simulink model "Main_EntryPoint"  (R2024b)
settings: Solver=VariableStepAuto  StartTime=0.0  StopTime=10.0  RelTol=1e-3
(part 2 of 2)

== stateflow chart Main_EntryPoint/Chart ==
  state Main_EntryPoint1 [parallel]
    Main_EntryPoint()
    settings: executionOrder=1
  data: i_byBlockDirectionId function_input uint8; i_stBlockDirectionData function_input Bus: ST_BlockDirection; staBlockDirectionAy temporary Bus: ST_BlockDirection size=8; o_stRegionData function_output Bus: ST_ShuntingRegionTable; i_byRegionId function_input uint8; i_staShuntingRegionArray function_input Bus: ST_ShuntingRegion size=16; stShuntingRegionData temporary Bus: ST_ShuntingRegion; i_byRegionId function_input BYTE; o_stRegionData function_output Bus: ST_MaintenanceRegion size=1; i_byRegionId function_input uint8; o_bResult function_output boolean; stTableData temporary Bus: ST_ShuntingRegionTable; i_byRegionId function_input BYTE; i_staRegionDataArray function_input Bus: ST_MaintenanceRegion size=16; o_stRegionData function_output Bus: ST_MaintenanceRegion; i_byShuntingId function_input BYTE; i_stShuntingData function_input Bus: ST_ShuntingRegion; i_byBlockDirectionId function_input uint8; i_stBlockDirectionData function_input Bus: ST_BlockDirection; i_staBlockDirectionArray function_input Bus: ST_BlockDirection size=8; o_staBlockDirectionArray function_output Bus: ST_BlockDirection size=8; i_byRegionId function_input uint8; i_staRegionArray function_input Bus: ST_ShuntingRegionTable size=16; o_stRegionData function_output Bus: ST_ShuntingRegionTable; i_staTableDataArray function_input Bus: ST_InterlockingTrackLock size=8; o_bResult function_output BOOL; o_bResult function_output BOOL; i_byRegionId function_input BYTE; i_byRegionId function_input BYTE; i_stRegionData function_input Bus: ST_ShuntingRegion; i_staShuntingRegionArray function_input Bus: ST_ShuntingRegion size=16; o_staShuntingRegionArray function_output Bus: ST_ShuntingRegion size=16; i_staTableDataArray function_input Bus: ST_InterlockingRouteCheck size=24; o_bResult function_output BOOL; i_byBlockDirectionId function_input uint8; i_bStatus function_input boolean; stBlockDirectionData temporary Bus: ST_BlockDirection; i_staTableDataArray function_input Bus: ST_InterlockingPointMachineCheck size=12; o_bResult function_output BOOL; i_byRegionId function_input uint8; o_bResult function_output BOOL; stRegionData temporary Bus: ST_MaintenanceRegion; i_byRegionId function_input BYTE; o_stRegionData function_output Bus: ST_ShuntingRegion; i_staTableDataArray function_input Bus: ST_InterlockingPointMachineCheck size=12; o_bResult function_output BOOL; i_byBlockDirectionId function_input BYTE; o_bResult function_output BOOL; i_staTableDataArray function_input Bus: ST_InterlockingRouteCheck size=24; o_bResult function_output BOOL; i_byRegionId function_input BYTE; i_staShuntingRegionArray function_input Bus: ST_ShuntingRegion size=16; o_stRegionData function_output Bus: ST_ShuntingRegion; i_staTableDataArray function_input Bus: ST_InterlockingSignalCheck size=8; o_bResult function_output BOOL; i_byBlockDirectionId function_input uint8; o_stBlockDirectionData function_output Bus: ST_BlockDirection; i_iType function_input INT; i_ID function_input BYTE; o_bIsCheckID function_output boolean; i_byRegionId function_input uint8; o_bResult function_output boolean; o_aLevelCrossingSetPowerAy function_output BOOL size=8; i_stCmd function_input Bus: ST_IXLCommand; stShuntingRegionTableData temporary Bus: ST_ShuntingRegionTable; i_byRegionId function_input uint8; o_IsExist function_output boolean; i_byBlockDirectionId function_input uint8; i_staBlockDirectionArray function_input Bus: ST_BlockDirection size=8; o_stBlockDirectionData function_output Bus: ST_BlockDirection; o_aPMSetNormalAy function_output BOOL size=36; o_aPMSetPowerAy function_output BOOL size=36; o_aPMSetReverseAy function_output BOOL size=36; i_byRegionId function_input uint8; o_bResult function_output boolean; i_byRegionId function_input uint8; o_bResult function_output boolean; i_bySignalId function_input BYTE; o_stSignalData function_output Bus: ST_Signal; o_aSignal1SetAy function_output BOOL size=36; o_aSignal2SetAy function_output BOOL size=36; o_aSignal3SetAy function_output BOOL size=36; o_aSignal4SetAy function_output BOOL size=36; i_byRegionId function_input uint8; o_bResult function_output boolean; stShuntingRegionData temporary Bus: ST_ShuntingRegion; i_byRegionId function_input BYTE; i_bySetCmd function_input BYTE; stShuntingRegionData temporary Bus: ST_ShuntingRegion; i_byRegionId function_input uint8; i_bySetStatus function_input uint8; stShuntingRegionData temporary Bus: ST_ShuntingRegion; i_byDataType function_input BYTE; i_byDataArray function_input BYTE size=8; o_bResult function_output BOOL; i_bySignalId function_input BYTE; i_staSignalArray function_input Bus: ST_Signal size=36; o_stSignalData function_output Bus: ST_Signal; i_byRegionId function_input BYTE; i_bSetSignalSign function_input BOOL; o_aStartPointAy function_output BOOL size=36; i_byDataType function_input BYTE; i_byDataArray function_input BYTE size=12; o_bResult function_output BOOL; i_byRoutingId function_input uint8; o_bResult function_output boolean; i_byStartPointId function_input uint8; o_bResult function_output boolean; i_byCrossingId function_input BYTE; o_bResult function_output BOOL; i_byTrackId function_input uint8; o_bResult function_output boolean; i_byDoorId function_input uint8; o_bResult function_output boolean; i_bySignalId function_input uint8; o_bResult function_output boolean; i_bCommandStatus function_input uint8; o_aTrackResetAy function_output BOOL size=48; i_byDataType function_input BYTE; i_byDataArray function_input BYTE size=24; o_bResult function_output BOOL; i_byRoutingId function_input BYTE; o_bResult function_output BOOL; i_bySignalId function_input uint8; o_bResult function_output boolean; stSignalData temporary Bus: ST_Signal; i_bCommandStatus function_input uint8; i_byDataType function_input BYTE; i_byDataId function_input BYTE; o_bResult function_output BOOL; i_byRoutingId function_input BYTE; o_stRoutingData function_output Bus: ST_Routing; i_byDataType function_input BYTE; o_iDataArrayLen function_output INT; i_uliErrorCodeUid function_input UDINT; i_bySignalId function_input BYTE; i_bySignalConfig function_input BYTE; i_bySignalSign function_input BYTE; stSignalData temporary Bus: ST_Signal; i_byRoutingId function_input BYTE; i_staRoutingArray function_input Bus: ST_Routing size=96; o_stRoutingData function_output Bus: ST_Routing; i_uliErrorCodeUid function_input UDINT; i_bySignalConfig function_input BYTE; o_bLight1 function_output BOOL; o_bLight2 function_output BOOL; o_bLight3 function_output BOOL; o_bLight4 function_output BOOL; i_byPointMachineId function_input uint8; o_stPointMachineData function_output Bus: ST_PointMachine; i_uliErrorCodeUid function_input UDINT; i_bySignalConfig function_input BYTE; i_staSignalTruthTableArray function_input Bus: ST_SignalTruthTable size=31; o_bLight1 function_output BOOL; o_bLight2 function_output BOOL; o_bLight3 function_output BOOL; o_bLight4 function_output BOOL; bySignalConfig temporary BYTE; i_byPointMachineId function_input uint8; i_staPointMachineArray function_input Bus: ST_PointMachine size=36; o_stPointMachineData function_output Bus: ST_PointMachine; i_uliErrorCodeUid function_input UDINT; i_bySignalId function_input BYTE; i_stSignalData function_input Bus: ST_Signal; i_byPointMachineId function_input uint8; i_byPointMachinePosition function_input uint8; o_bResult function_output boolean; i_uliErrorCodeUid function_input UDINT; i_byType function_input BYTE; i_byPointMachineId function_input uint8; o_bResult function_output boolean; i_bySignalId function_input BYTE; i_stSignalData function_input Bus: ST_Signal; i_staSignalArray function_input Bus: ST_Signal size=36; o_staSignalArray function_output Bus: ST_Signal size=36; g_stStatusCode data_store_memory; g_stArrayLens data_store_memory; g_stSystemValue local double; g_stErrorCode data_store_memory; g_staErrorData data_store_memory; g_staShuntingRegionTable data_store_memory; g_staSendBlockDirection data_store_memory; g_staLevelCrossing data_store_memory; g_staMaintenanceRegion data_store_memory; g_staPlatformDoor data_store_memory; g_staPointMachine data_store_memory; g_staRouting data_store_memory; g_staSignal data_store_memory; g_staStartPoint data_store_memory; g_staTrack data_store_memory; g_staSignalTruthTable data_store_memory; g_staShuntingRegion data_store_memory; g_stExecuteIXLCommand data_store_memory; g_stSystemMonitor data_store_memory; g_stCheckType data_store_memory; g_stDOModuleAdapter data_store_memory; g_stOpcuaAdapter data_store_memory
  function BlockDirection_Set(i_byBlockDirectionId, i_stBlockDirectionData):
    | function BlockDirection_Set(i_byBlockDirectionId, i_stBlockDirectionData)
    |     
    |     global g_staSendBlockDirection;    
    | 
    |     % Set the block direction data
    |     staBlockDirectionAy = BlockDirection_SetData(i_byBlockDirectionId, i_stBlockDirectionData, g_staSendBlockDirection);
    | 
    |     % Copy the array
    |     g_staSendBlockDirection = staBlockDirectionAy;
    | end
  function o_stRegionData = CheckTable_GetShunting(i_byRegionId):
    | function o_stRegionData = CheckTable_GetShunting(i_byRegionId)
    | global g_staShuntingRegionTable;
    |     o_stRegionData = CheckTable_GetShuntingData(i_byRegionId, g_staShuntingRegionTable);
    | end
  function Shunting_Init(i_staShuntingRegionArray):
    | function Shunting_Init(i_staShuntingRegionArray)
    |     global g_stStatusCode;
    |     global g_stArrayLens;
    |     % Initialize variables
    |     iIndex = g_stStatusCode.INTDefault;
    |     byShuntingRegionId = g_stStatusCode.BYTEDefault;
    |     
    |     % Loop through the shunting region array
    |     for iIndex = g_stArrayLens.StartIndex:(g_stArrayLens.ShuntingRegionArrayLen - 1)
    |         byShuntingRegionId = i_staShuntingRegionArray(iIndex + 1).byShuntingRegionId;
    | 
    |         if byShuntingRegionId > g_stStatusCode.MinimumID
    |             % Get the shunting region data
    |             stShuntingRegionData = i_staShuntingRegionArray(iIndex + 1);
    |             % Set the status to initialized
    |             stShuntingRegionData.byStatus = g_stStatusCode.ShuntingRegionStatusInit;
    |             % Set the shunting region data
    |             Shunting_Set(byShuntingRegionId, stShuntingRegionData);
    |         else
    |             % Invalid ID, do nothing
    |         end
    |     end
    | end
  function o_stRegionData = Maintenance_Get(i_byRegionId):
    | function o_stRegionData = Maintenance_Get(i_byRegionId)
    |     global g_staMaintenanceRegion;
    |     o_stRegionData = Maintenance_GetData(i_byRegionId, g_staMaintenanceRegion);
    | 
    | end
  function o_bResult = CheckData_CheckShuntingRegionTableData(i_byRegionId):
    | function o_bResult = CheckData_CheckShuntingRegionTableData(i_byRegionId)
    |     global g_stStatusCode;
    |     global g_stErrorCode;
    |     global g_stArrayLens;
    |     % Initialize the output result
    |     o_bResult = true;
    | 
    |     % Initialize variables
    |     iIndex = g_stStatusCode.INTDefault;
    |     bySignalId = g_stStatusCode.BYTEDefault;
    |     bIsShuntingTableExist = false;
    |     bIsShuntingExist = false;
    |     bIsPointMachineCheckExist = false;
    |     bIsTrackCheckOSExist = false;
    |     bIsTrackCheckPlatformExist = false;
    |     bIsRouteCheckInSetExist = false;
    |     bIsSignalExist = false;
    |     
    | 
    |     % Check if shunting table exists
    |     bIsShuntingTableExist = CheckTable_IsShuntingTableExit(i_byRegionId);
    | 
    |     if bIsShuntingTableExist
    |         % Get shunting table data
    |         stTableData = CheckTable_GetShunting(i_byRegionId);
    | 
    |         % Check if shunting exists
    |         bIsShuntingExist = Shunting_IsExist(i_byRegionId);
    | 
    |         % Check interlocking point machine existence
    |         bIsPointMachineCheckExist = CheckData_CheckInterlockingPointMachineExistLen12(stTableData.PointMachineCheckArray);
    | 
    |         % Check interlocking track lock existence for OS array
    |         bIsTrackCheckOSExist = CheckData_CheckInterlockingTrackLockExistLen8(stTableData.TrackCheckOSArray);
    | 
    |         % Check interlocking track lock existence for platform array
    |         bIsTrackCheckPlatformExist = CheckData_CheckInterlockingTrackLockExistLen8(stTableData.TrackCheckPlatformArray);
    | 
    |         % Check interlocking route existence
    |         bIsRouteCheckInSetExist = CheckData_CheckInterlockingRouteExistLen24(stTableData.RouteCheckInSetArray);
    | 
    |         % Check if all conditions are met
    |         if bIsShuntingExist && bIsPointMachineCheckExist && bIsTrackCheckOSExist && bIsTrackCheckPlatformExist && bIsRouteCheckInSetExist
    |             % All arrays exist
    |         else
    |             o_bResult = false;
    |             SystemMonitor_SetWarningLog(g_stErrorCode.BM20_02_202);
    |         end
    | 
    |         % Loop through the signal check array
    |         for iIndex = g_stArrayLens.StartIndex:(stTableData.SignalCheckArrayLen - 1)
    |             bySignalId = stTableData.SignalCheckArray(iIndex + 1).bySignalId;
    | 
    |             if bySignalId > g_stStatusCode.MinimumID
    |                 % Check if signal exists
    |                 bIsSignalExist = Signal_IsExist(bySignalId);
    | 
    |                 if bIsSignalExist
    |                     % Signal exists
    |                 else
    |                     o_bResult = false;
    |                     SystemMonitor_SetWarningLog(g_stErrorCode.BM20_03_202);
    |                 end
    |             else
    |                 % ID not match
    |             end
    |         end
    |     else
    |         o_bResult = false;
    |         SystemMonitor_SetWarningLog(g_stErrorCode.BM20_01_202);
    |     end
    | end
  function Main_EntryPoint:
    | function Main_EntryPoint
    | global g_stStatusCode;
    | global g_stSystemValue
    | 
    | Main_InitProcess();
    |  
    | if g_stSystemValue.byProgramStatus == g_stStatusCode.SystemValueProgramStatusNormal
    |     Main_SystemNormal();
    | else
    |     Main_SystemException();
    | end
  function o_stRegionData = Maintenance_GetData(i_byRegionId, i_staRegionDataArray):
    | function o_stRegionData = Maintenance_GetData(i_byRegionId, i_staRegionDataArray)
    |     global g_stStatusCode;
    |     global g_stArrayLens;
    |    
    |      o_stRegionData = i_staRegionDataArray(1);
    |     % 檢查區域 ID 是否大於最小 ID
    |     if i_byRegionId > g_stStatusCode.MinimumID
    |         % 遍歷陣列以查找匹配的區域 ID
    |         for iIndex = g_stArrayLens.StartIndex:g_stArrayLens.MaintenanceRegionArrayLen - 1
    |             if i_byRegionId == i_staRegionDataArray(iIndex + 1).byMaintenanceRegionId
    |                 o_stRegionData = i_staRegionDataArray(iIndex + 1);
    |                 return;
    |             end
    |         end
    |     else
    |    
    |     end
    | 
    |  
    | end
  function Main_InitProcess:
    | function Main_InitProcess
    |     global g_stSystemValue;
    |     global g_stStatusCode;
    |     % Check if the system is not initialized
    |     if g_stSystemValue.IsInit == g_stStatusCode.SystemValueIsInitNon
    |         % Initialize the main object
    |         Main_InitObject();
    | 
    |         % Set the system initialization status to done
    |         g_stSystemValue.IsInit = g_stStatusCode.SystemValueIsInitDone;
    |     else
    |         % Do nothing if already initialized
    |     end
    | end
  function Main_InitObject:
    | function Main_InitObject
    |     % Initialize various components
    |     % BlockDirection_Init(SendBlockDirectionArray);
    |     % LevelCrossing_Init(LevelCrossingArray);
    |     % Maintenance_Init(MaintenanceRegionArray);
    |     % PlatformDoor_Init(PlatformDoorArray);
    |     % PointMachine_Init(PointMachineArray);
    |     % Routing_Init(RoutingArray);
    |     Shunting_Init(g_staShuntingRegion);
    |     % Signal_Init(SignalArray);
    |     % StartPoint_Init(StartPointArray);
    |     % Track_Init(TrackArray);
    |     % SystemMonitor_Init();
    | end
  function Shunting_Set(i_byShuntingId, i_stShuntingData):
    | function Shunting_Set(i_byShuntingId, i_stShuntingData)
    |     
    | global g_staShuntingRegion;    
    | 
    |     % Set the block direction data
    |     staShuntingAy = Shunting_SetData(i_byShuntingId, i_stShuntingData, g_staShuntingRegion);
    | 
    |     % Copy the array
    |     g_staShuntingRegion = staShuntingAy;
    | end
  function o_staBlockDirectionArray = BlockDirection_SetData(i_byBlockDirectionId, i_stBlockDirectionData, i_staBlockDirectionArray):
    | function o_staBlockDirectionArray = BlockDirection_SetData(i_byBlockDirectionId, i_stBlockDirectionData, i_staBlockDirectionArray)
    |     global g_stStatusCode;
    |     global g_stArrayLens;
    |     
    |     % Initialize the index
    |     %iIndex = g_stStatusCode.INTDefault;
    | 
    |     % Copy the input array to the output array
    |     o_staBlockDirectionArray = i_staBlockDirectionArray;
    | 
    |     % Check if the block direction ID is valid
    |     if i_byBlockDirectionId > g_stStatusCode.MinimumID
    |         % Loop through the block direction array
    |         for iIndex = g_stArrayLens.StartIndex:g_stArrayLens.SendBlockDirectionArrayLen - 1
    |             % Check if the current block direction ID matches the input ID
    |             if i_byBlockDirectionId == o_staBlockDirectionArray(iIndex + 1).byBlockDirectionId
    |                 % Update the matching block direction data
    |                 o_staBlockDirectionArray(iIndex + 1) = i_stBlockDirectionData;
    |             else
    |                 % Not equal ID, do nothing
    |             end
    |         end
    |     else
    |         % Invalid ID, do nothing
    |     end
    | end
  function o_stRegionData = CheckTable_GetShuntingData(i_byRegionId, i_staRegionArray):
    | function o_stRegionData = CheckTable_GetShuntingData(i_byRegionId, i_staRegionArray)
    |     global g_stStatusCode;
    |     global g_stArrayLens;
    |     % 初始化索引和區域 ID
    |     iIndex = g_stStatusCode.INTDefault;
    |     byRegionId = g_stStatusCode.BYTEDefault;
    | 
    |     o_stRegionData = i_staRegionArray(1);
    |     % 檢查區域 ID 是否大於最小 ID
    |     if i_byRegionId > g_stStatusCode.MinimumID
    |         % 遍歷陣列以查找匹配的區域 ID
    |         for iIndex = g_stArrayLens.StartIndex:g_stArrayLens.ShuntingRegionTableArrayLen - 1
    |             byRegionId = i_staRegionArray(iIndex + 1).byShuntingRegionId;
    | 
    |             if byRegionId == i_byRegionId
    |                 o_stRegionData = i_staRegionArray(iIndex + 1);
    |                 return;
    |             end
    |         end
    |     else
    |        
    |     end
    | 
    | end
  function Main_SystemNormal:
    | function Main_SystemNormal
    | 
    | %Porcess
    | Main_DispatchClientCommand();
    | 
    | end
  function o_bResult = CheckData_CheckInterlockingTrackLockExistLen8(i_staTableDataArray):
    | function o_bResult = CheckData_CheckInterlockingTrackLockExistLen8(i_staTableDataArray)
    |     global g_stArrayLens;
    |     global g_stStatusCode;
    |     global g_stErrorCode;
    |    
    |     % Initialize variables
    |     o_bResult = true;
    |     iIndex = g_stStatusCode.INTDefault;
    |     byTrackId = g_stStatusCode.BYTEDefault;
    |     bIsTrackExist = false;
    | 
    |     % Loop through the input array
    |     for iIndex = g_stArrayLens.StartIndex : g_stArrayLens.ArrayLen8 -1
    |         byTrackId = i_staTableDataArray(iIndex + 1).byTrackId;
    | 
    |         % Check if the track ID is valid
    |         if byTrackId > g_stStatusCode.MinimumID
    |             % Check if the track exists
    |             bIsTrackExist = Track_IsExist(byTrackId);
    | 
    |             % If the track does not exist, set the result to false and log a warning
    |             if ~bIsTrackExist
    |                 o_bResult = false;
    |                 SystemMonitor_SetWarningLog(g_stErrorCode.BM14_01_202);
    |             end
    |         end
    |     end
    | end
  function o_bResult = Maintenance_IsExist(i_byRegionId):
    | function o_bResult = Maintenance_IsExist(i_byRegionId)
    |   global g_stStatusCode;
    |   o_bResult = CheckData_CheckDataExist(g_stStatusCode.DataTypeMaintenance, i_byRegionId);
    | end
  function o_staShuntingRegionArray = Shunting_SetData(i_byRegionId, i_stRegionData, i_staShuntingRegionArray):
    | function o_staShuntingRegionArray = Shunting_SetData(i_byRegionId, i_stRegionData, i_staShuntingRegionArray)
    |     global g_stStatusCode;
    |     global g_stArrayLens;
    |     % Initialize the index
    |    
    |     o_staShuntingRegionArray = i_staShuntingRegionArray;
    |     % Check if the region ID is valid
    |     if i_byRegionId > g_stStatusCode.MinimumID
    |         % Loop through the shunting region array
    |         for iIndex = g_stArrayLens.StartIndex:(g_stArrayLens.ShuntingRegionArrayLen - 1)
    |             if i_byRegionId == o_staShuntingRegionArray(iIndex + 1).byShuntingRegionId
    |                 % Update the shunting region data
    |                 o_staShuntingRegionArray(iIndex + 1) = i_stRegionData;
    |             else
    |                 % Not equal ID, do nothing
    |             end
    |         end
    |     else
    |         % Invalid ID, do nothing
    |     end
    | end
  function o_bResult = CheckTable_CheckInterlockingRouteCheckExecuteLen24(i_staTableDataArray):
    | function o_bResult = CheckTable_CheckInterlockingRouteCheckExecuteLen24(i_staTableDataArray)
    |     global g_stArrayLens;
    |     global g_stStatusCode;
    | 
    |     % Initialize variables
    |     o_bResult = false;
    |     iIndex = g_stStatusCode.INTDefault;
    |     byRouteId = g_stStatusCode.BYTEDefault;
    |     bIsExecute = false;
    | 
    |     % Loop through the array
    |     for iIndex = g_stArrayLens.StartIndex:(g_stArrayLens.ArrayLen24 - 1)
    |         byRouteId = i_staTableDataArray(iIndex).byRouteId;
    | 
    |         if byRouteId > g_stStatusCode.MinimumID
    |             bIsExecute = Routing_IsExecute(byRouteId);
    | 
    |             if bIsExecute
    |                 o_bResult = true;
    |                 % SystemMonitor_SetSafeLog(g_stErrorCode.BA13_01_207);
    |             else
    |                 % Routing not execute
    |                 % SystemMonitor_SetSafeLog(g_stErrorCode.BA13_02_208);
    |             end
    |         else
    |             % ID not match
    |         end
    |     end
    | end
  function BlockDirection_SetShunting(i_byBlockDirectionId, i_bStatus):
    | function BlockDirection_SetShunting(i_byBlockDirectionId, i_bStatus)
    |     
    |     % 检查 ID 是否有效
    |     if i_byBlockDirectionId > g_stStatusCode.MinimumID
    |         % 获取 BlockDirection 数据
    |         stBlockDirectionData = BlockDirection_Get(i_byBlockDirectionId);
    | 
    |         % 更新结构体数据
    |         stBlockDirectionData.bSetShuntingRegion = i_bStatus;
    | 
    |         % 重新设置 BlockDirection
    |         BlockDirection_Set(i_byBlockDirectionId, stBlockDirectionData);
    |     else
    | 
    |     end
    | end
  function Main_SystemException:
    | function Main_SystemException
    | %/*Input*/
    | Main_UpdateSystemValue();
    | % /* Main___ProcessDigitalInput(); */
    | 
    | % /*Porcess don't work*/
    | 
    | % /*Output*/
    | SystemMonitor_SetDigitalOutputFault();
    | 
    | %/ *待開發中還，在QT沒想好怎麼寫*/
    | %SystemMonitor_SetSafeEthernetOutputFault(); 
    | 
    | Main_ReportSystemStatus();
    | end
  function o_bResult = CheckData_CheckInterlockingPointMachineExistLen12(i_staTableDataArray):
    | function o_bResult = CheckData_CheckInterlockingPointMachineExistLen12(i_staTableDataArray)
    |     global g_stArrayLens;
    |     global g_stStatusCode;
    |     global g_stErrorCode;
    |    
    |     % Initialize variables
    |     o_bResult = true;
    |     iIndex = g_stStatusCode.INTDefault;
    |     byPointMachineId = g_stStatusCode.BYTEDefault;
    |     bIsPointMachineExist = false;
    | 
    |     % Loop through the input array
    |     for iIndex = g_stArrayLens.StartIndex : g_stArrayLens.ArrayLen12 -1
    | 
    |         byPointMachineId = i_staTableDataArray(iIndex + 1).byPointMachineId;
    | 
    |         byPointMachinePosition = i_staTableDataArray(iIndex + 1).byPointMachinePosition;
    | 
    |         % Check if the track ID is valid
    |         if byPointMachineId > g_stStatusCode.MinimumID && byPointMachinePosition > g_stStatusCode.MinimumID
    |             % Check if the track exists
    |             bIsPointMachineExist = PointMachine_IsExist(byPointMachineId);
    | 
    |             % If the track does not exist, set the result to false and log a warning
    |             if ~bIsPointMachineExist
    |                 o_bResult = false;
    |                 SystemMonitor_SetWarningLog(g_stErrorCode.BM15_01_202);
    |             end
    |         end
    |     end
    | end
  function o_bResult = Maintenance_IsSet(i_byRegionId):
    | function o_bResult = Maintenance_IsSet(i_byRegionId)
    |     global g_stStatusCode;
    |     % 初始化結果為 false
    |     o_bResult = false;
    | 
    |     % 獲取區域數據
    |     stRegionData = Maintenance_Get(i_byRegionId);
    | 
    |     % 檢查區域的狀態
    |     if stRegionData.byStatus == g_stStatusCode.IsStatusUnSet
    |         % Maintenance 未設置
    |         o_bResult = false;
    |     elseif stRegionData.byStatus == g_stStatusCode.IsStatusSet
    |         % Maintenance 已設置
    |         o_bResult = true;
    |     else
    |         % 其他狀態視為未設置
    |         o_bResult = false;
    |     end
    | end
  function SystemMonitor_UpdateSystemTime:
    | function SystemMonitor_UpdateSystemTime
    |  global g_stSystemValue;
    |  global g_stSystemMonitor;
    |     g_stSystemValue.Timestamp_ms = g_stSystemMonitor.HardwareValue.Timestamp_ms;
    | 
    |     g_stSystemValue.Timestamp_sec = g_stSystemMonitor.HardwareValue.Timestamp_sec;
    | end
  function Main_UpdateSystemValue:
    | function Main_UpdateSystemValue()
    |     global g_stSystemValue;
    |     global g_stSystemMonitor;
    | 
    |     % Update the system time
    |     SystemMonitor_UpdateSystemTime();
    | 
    |     % Get the current date and time
    |     
    | 
    |     % Update the timestamp values
    |     g_stSystemValue.Timestamp_ms = g_stSystemMonitor.HardwareValue.Timestamp_ms;
    |     g_stSystemValue.Timestamp_sec = g_stSystemMonitor.HardwareValue.Timestamp_sec;
    | 
    |     % Reset the error log
    |     SystemMonitor_ResetErrorLog();
    | end
  function Main_DispatchClientCommand:
    | function Main_DispatchClientCommand
    | global g_stCheckType;
    | global g_stStatusCode
    | global g_stExecuteIXLCommand;
    | 
    | 
    | 
    | 
    | 
    | global g_stErrorCode;
    |     % Initialize the check ID flag Terry
    |     bIsCheckID = false;
    | 
    |     % Execute the IXL command (assuming ExecuteIXLCommand is a function)
    |     stIXLCommand = g_stExecuteIXLCommand;
    | 
    |     % Check the ID
    |     bIsCheckID = CheckID(g_stCheckType.MinID, stIXLCommand.byCommand);
    | 
    |     % Process the command if the ID check is true
    |     if bIsCheckID
    |         if stIXLCommand.byStatus == g_stStatusCode.IXLCmdStatusInit || ...
    |            stIXLCommand.byStatus == g_stStatusCode.IXLCmdStatusExecuting
    |             if stIXLCommand.byCommand == g_stStatusCode.IXLCommandSetRoute
    |                 SetShunting_Command(stIXLCommand);
    |             % if stIXLCommand.byCommand == g_stStatusCode.IXLCommandSetRoute
    |             %     SetRoute_Command(stIXLCommand);
    |             % elseif stIXLCommand.byCommand == g_stStatusCode.IXLCommandCancelRoute
    |             %     CancelRoute_Command(stIXLCommand);
    |             % elseif stIXLCommand.byCommand == g_stStatusCode.IXLCommandResetTrack
    |             %     ResetTrack_Command(stIXLCommand);
    |             % elseif stIXLCommand.byCommand == g_stStatusCode.IXLCommandTurnPM
    |             %     TurnPM_Command(stIXLCommand);
    |             % elseif stIXLCommand.byCommand == g_stStatusCode.IXLCommandSetMaintenance
    |             %     SetMaintenance_Command(stIXLCommand);
    |             % elseif stIXLCommand.byCommand == g_stStatusCode.IXLCommandResetMaintenance
    |             %     ResetMaintenance_Command(stIXLCommand);
    |             % elseif stIXLCommand.byCommand == g_stStatusCode.IXLCommandSetShunting
    |             %     SetShunting_Command(stIXLCommand);
    |             % elseif stIXLCommand.byCommand == g_stStatusCode.IXLCommandResetShunting
    |             %     ResetShunting_Command(stIXLCommand);
    |             % elseif stIXLCommand.byCommand == g_stStatusCode.IXLCommandSetBlockade
    |             %     SetBlockade_Command(stIXLCommand);
    |             % elseif stIXLCommand.byCommand == g_stStatusCode.IXLCommandResetBlockade
    |             %     ResetBlockade_Command(stIXLCommand);
    |             else
    |                 %亂給的輸入
    |                 SystemMonitor_SetProgramException(g_stErrorCode.BM20_01_202);
    |             end
    |         end
    |     end
    | end
  function o_stRegionData = Shunting_Get(i_byRegionId):
    | function o_stRegionData = Shunting_Get(i_byRegionId)
    | global g_staShuntingRegion;
    |     o_stRegionData = Shunting_GetData(i_byRegionId, g_staShuntingRegion);
    | 
    | end
  function o_bResult = CheckTable_CheckInterlockingPointMachineCheckPositionLen12(i_staTableDataArray):
    | function o_bResult = CheckTable_CheckInterlockingPointMachineCheckPositionLen12(i_staTableDataArray)
    |     global g_stArrayLens;
    |     global g_stStatusCode;
    | 
    |     % Initialize variables
    |     o_bResult = true;
    |     iIndex = g_stStatusCode.INTDefault;
    |     byPointMachineId = g_stStatusCode.BYTEDefault;
    |     byPointMachinePosition = g_stStatusCode.BYTEDefault;
    |     bIsPositionCorrect = false;
    | 
    |     % Loop through the array
    |     for iIndex = g_stArrayLens.StartIndex:(g_stArrayLens.ArrayLen12 - 1)
    |         byPointMachineId = i_staTableDataArray(iIndex).byPointMachineId;
    |         byPointMachinePosition = i_staTableDataArray(iIndex).byPointMachinePosition;
    | 
    |         if byPointMachineId > g_stStatusCode.MinimumID
    |             bIsPositionCorrect = PointMachine_IsPositionCorrect(byPointMachineId, byPointMachinePosition);
    | 
    |             if byPointMachinePosition == g_stStatusCode.PointMachinePositionNotCheck
    |                 % UnCheck position
    |                 % SystemMonitor_SetWarningLog(g_stErrorCode.BA09_03_215);
    |             elseif ~bIsPositionCorrect
    |                 o_bResult = false;
    |                 % SystemMonitor_SetWarningLog(g_stErrorCode.BA09_01_214);
    |             else
    |                 % TurnPM position is valid
    |             end
    |         else
    |             % ID not match
    |         end
    |     end
    | end
  function o_bResult = BlockDirection_IsExist(i_byBlockDirectionId):
    | function o_bResult = BlockDirection_IsExist(i_byBlockDirectionId)
    |     global g_stStatusCode;
    |     o_bResult = CheckData_CheckDataExist(g_stStatusCode.DataTypeBlockDirection, i_byBlockDirectionId);
    |   
    | end
  function Main_ReportSystemStatus:
    | function Main_ReportSystemStatus()
    | 
    | % QT建立一半而已，還沒補
    | % ReportMonitor_DIModule();
    | % 
    | % ReportMonitor_DOModule();
    | % 
    | % ReportMonitor_SystemModule();
    | %
    |     ReportMonitor_SystemValue();
    | % 
    |     ReportObject_MaintenanceRegionST();
    | %
    |     ReportObject_PointMachineST();
    | % 
    |     ReportObject_RoutingST();
    | % 
    |     ReportObject_ShuntingRegionST();
    | % 
    |     ReportObject_SignalST();
    | % 
    |     ReportObject_TrackST();
    | 
    | end
  function o_bResult = CheckData_CheckInterlockingRouteExistLen24(i_staTableDataArray):
    | function o_bResult = CheckData_CheckInterlockingRouteExistLen24(i_staTableDataArray)
    |     global g_stArrayLens;
    |     global g_stStatusCode;
    |     global g_stErrorCode;
    |    
    |     % Initialize variables
    |     o_bResult = true;
    |     iIndex = g_stStatusCode.INTDefault;
    |     byRouteId = g_stStatusCode.BYTEDefault;
    |     bIsRoutingExist = false;
    | 
    |     % Loop through the input array
    |     for iIndex = g_stArrayLens.StartIndex : g_stArrayLens.ArrayLen24 -1
    | 
    |         byRouteId = i_staTableDataArray(iIndex + 1).byRouteId;
    | 
    |         % Check if the track ID is valid
    |         if byRouteId > g_stStatusCode.MinimumID
    |             % Check if the track exists
    |             bIsRoutingExist = Routing_IsExist(byRouteId);
    | 
    |             % If the track does not exist, set the result to false and log a warning
    |             if ~bIsRoutingExist
    |                 o_bResult = false;
    |                 SystemMonitor_SetWarningLog(g_stErrorCode.BM16_01_202);
    |             end
    |         end
    |     end
    | end
  function SystemMonitor_SetDigitalOutputFault:
    | function SystemMonitor_SetDigitalOutputFault()
    | global g_stDOModuleAdapter;
    |     % Set level crossing fault
    |     g_stDOModuleAdapter.bSetLevelCrossingPowerAy = SystemMonitor_SetLevelCrossingFault();
    | 
    |     % Set point machine fault
    |     g_stDOModuleAdapter.bPMSetNormalAy, ...
    |     g_stDOModuleAdapter.bPMSetPowerAy, ...
    |     g_stDOModuleAdapter.bPMSetReverseAy = SystemMonitor_SetPointMachineFault();
    | 
    |     % Set signal fault
    |     g_stDOModuleAdapter.bSignal1SetAy, ...
    |     g_stDOModuleAdapter.bSignal2SetAy, ...
    |     g_stDOModuleAdapter.bSignal3SetAy, ...
    |     g_stDOModuleAdapter.bSignal4SetAy = SystemMonitor_SetSignalFault();
    | 
    |     % Set start point fault
    |     g_stDOModuleAdapter.bStartPointAy = SystemMonitor_SetStartPointFault();
    | 
    |     % Set track fault
    |     g_stDOModuleAdapter.bTrackResetAy = SystemMonitor_SetTrackFault();
    | end
  function o_stRegionData = Shunting_GetData(i_byRegionId, i_staShuntingRegionArray):
    | function o_stRegionData = Shunting_GetData(i_byRegionId, i_staShuntingRegionArray)
    |     global g_stStatusCode;
    |     global g_stArrayLens;
    | 
    |      o_stRegionData=i_staShuntingRegionArray(1);
    |     % 檢查區域 ID 是否大於最小 ID
    |     if i_byRegionId > g_stStatusCode.MinimumID
    |         % 遍歷陣列以查找匹配的區域 ID
    |         for iIndex = g_stArrayLens.StartIndex:g_stArrayLens.ShuntingRegionArrayLen - 1
    |             if i_byRegionId == i_staShuntingRegionArray(iIndex + 1).byShuntingRegionId
    |                 o_stRegionData = i_staShuntingRegionArray(iIndex + 1);
    |                 return;
    |             end
    |         end
    |     else
    |         
    |     end
    | 
    | end
  function o_bResult = CheckTable_CheckInterlockingSignalCheckLockLen8(i_staTableDataArray):
    | function o_bResult = CheckTable_CheckInterlockingSignalCheckLockLen8(i_staTableDataArray)
    | global g_stArrayLens;
    | global g_stStatusCode;
    |     % Initialize variables
    |     o_bResult = false;
    |     iIndex = g_stStatusCode.INTDefault;
    |     bIsSignalLock = false;
    |     bySignalId = g_stStatusCode.BYTEDefault;
    | 
    |     % Loop through the array
    |     for iIndex = g_stArrayLens.StartIndex:(g_stArrayLens.ArrayLen8 - 1)
    |         bySignalId = i_staTableDataArray(iIndex).bySignalId;
    | 
    |         if bySignalId > g_stStatusCode.MinimumID
    |             bIsSignalLock = Signal_IsLock(bySignalId);
    | 
    |             if bIsSignalLock
    |                 o_bResult = true;
    | 
    |                 % SystemMonitor___SetSafeLog(g_stErrorCode.BA20_01_203);
    |             else
    |                 % Signal isn't locked
    | 
    |                 % SystemMonitor___SetSafeLog(g_stErrorCode.BA20_02_204);
    |             end
    |         else
    |             % ID not match
    |         end
    |     end
    | end
  function o_stBlockDirectionData = BlockDirection_Get(i_byBlockDirectionId):
    | function o_stBlockDirectionData = BlockDirection_Get(i_byBlockDirectionId)
    | global g_staSendBlockDirection;
    |     o_stBlockDirectionData = BlockDirection_GetData(i_byBlockDirectionId, g_staSendBlockDirection);
    | end
  function o_bIsCheckID = CheckID(i_iType, i_ID):
    | function o_bIsCheckID = CheckID(i_iType, i_ID)
    |     global g_stStatusCode;
    |     global g_stCheckType;
    |     %global CheckType
    |     % Initialize the output flag
    |     o_bIsCheckID = false;
    | 
    |     % Check if the type matches g_stCheckType.MinID
    |     if i_iType == g_stCheckType.MinID
    |         % Check if the ID is greater than g_stStatusCode.MinimumID
    |         if g_stStatusCode.MinimumID < i_ID
    |             o_bIsCheckID = true;
    |         else
    |             o_bIsCheckID = false;
    |         end
    |     else
    |         o_bIsCheckID = false;
    |     end
    | end
  function o_bResult = Shunting_IsExist(i_byRegionId):
    | function o_bResult = Shunting_IsExist(i_byRegionId)
    | global g_stStatusCode
    |     % Call the CheckData_CheckDataExist function with the shunting data type and region ID
    |     o_bResult = CheckData_CheckDataExist(g_stStatusCode.DataTypeShunting, i_byRegionId);
    | end
  function o_aLevelCrossingSetPowerAy = SystemMonitor_SetLevelCrossingFault:
    | function o_aLevelCrossingSetPowerAy = SystemMonitor_SetLevelCrossingFault()
    | global g_stStatusCode;
    | global g_stArrayLens;
    | global g_stDOModuleAdapter;
    |     % Initialize the index
    |     iIndex = g_stStatusCode.INTDefault;
    |     o_aLevelCrossingSetPowerAy = false(8, 1);
    |     % Loop through the LevelCrossingArray
    |     for iIndex = g_stArrayLens.StartIndex:g_stArrayLens.LevelCrossingArrayLen - 1
    |         % Check if the index is within the bounds of SetLevelCrossingPowerAyLen
    |         if iIndex < g_stDOModuleAdapter.SetLevelCrossingPowerAyLen
    |             % Set the corresponding element to IsUnSet
    |             o_aLevelCrossingSetPowerAy(iIndex + 1) = g_stStatusCode.IsUnSet;
    |         else
    |             % Do nothing if the index is out of bounds
    |         end
    |     end
    | end
  function SetShunting_Command(i_stCmd):
    | function SetShunting_Command(i_stCmd)
    |     global g_stStatusCode;
    |     global g_stErrorCode;
    |     
    |     % Initialize variables
    |     bIsCheckSetData = false;
    |     bIsShuntingSet = false;
    |     bIsMaintenanceSet = false;
    |     bIsRouteExecute = false;
    |     bCheckTurnPMPosition = false;
    |     bIsSignalLock = false;
    |     byRegionId = g_stStatusCode.BYTEDefault;
    | 
    | 
    |     % Get the region ID from the command
    |     byRegionId = i_stCmd.byCmd_SetShunting_RegionId;
    | 
    |     % Check set data
    |     bIsCheckSetData = SetShunting_CheckSetData(byRegionId);
    | 
    |     if bIsCheckSetData
    |         % Check if shunting is set
    |         bIsShuntingSet = Shunting_IsSet(byRegionId);
    | 
    |         % Check if maintenance is set
    |         bIsMaintenanceSet = Maintenance_IsSet(byRegionId);
    | 
    |         if ~bIsShuntingSet && ~bIsMaintenanceSet
    |             % Get shunting region table data
    |             stShuntingRegionTableData = CheckTable_GetShunting(byRegionId);
    |          
    |             % Check interlocking route execute
    |             bIsRouteExecute = CheckTable_CheckInterlockingRouteCheckExecuteLen24(stShuntingRegionTableData.RouteCheckInSetArray);
    | 
    |             % Check interlocking point machine check position
    |             bCheckTurnPMPosition = CheckTable_CheckInterlockingPointMachineCheckPositionLen12(stShuntingRegionTableData.PointMachineCheckArray);
    | 
    |             % Check interlocking signal check lock
    |             bIsSignalLock = CheckTable_CheckInterlockingSignalCheckLockLen8(stShuntingRegionTableData.SignalCheckArray);
    | 
    |             if ~bIsRouteExecute && bCheckTurnPMPosition && ~bIsSignalLock
    |                 % Set shunting status
    |                 SetShunting_SetStatus(byRegionId, g_stStatusCode.IsStatusSet);
    | 
    |                 % Complete the command
    |                 CommonCommand_Complete(g_stStatusCode.IXLCmdStatusSuccess);
    | 
    |                 % Set safe log
    |                 SystemMonitor_SetSafeLog(g_stErrorCode.AH02_04_003);
    |             else
    |                 % Discard the command
    |                 CommonCommand_Discard(g_stStatusCode.IXLCmdStatusFailToCheckInterlockingTable);
    | 
    |                 % Set warning log
    |                 SystemMonitor_SetWarningLog(g_stErrorCode.AH02_03_005);
    |             end
    |         else
    |             % Discard the command
    |             CommonCommand_Discard(g_stStatusCode.IXLCmdStatusSetRegionFault);
    | 
    |             % Set warning log
    |             SystemMonitor_SetWarningLog(g_stErrorCode.AH02_02_009);
    |         end
    |     else
    |         % Discard the command
    |         CommonCommand_Discard(g_stStatusCode.IXLCmdStatusFailToQueryInterlockingTable);
    | 
    |         % Set program exception
    |         SystemMonitor_SetProgramException(g_stErrorCode.AH02_01_004);
    |     end
    | end
  function o_IsExist = CheckTable_IsShuntingTableExit(i_byRegionId):
    | function o_IsExist = CheckTable_IsShuntingTableExit(i_byRegionId)
    |     global g_stStatusCode;
    |     global g_stArrayLens;
    |     global g_staShuntingRegionTable;
    |     % Initialize variables
    |     o_IsExist = false;
    |     iIndex = g_stStatusCode.INTDefault;
    |     byRegionId = g_stStatusCode.BYTEDefault;
    | 
    |     % Loop through the ShuntingRegionTableArray
    |     for iIndex = g_stArrayLens.StartIndex:g_stArrayLens.ShuntingRegionTableArrayLen - 1
    |         byRegionId = g_staShuntingRegionTable(iIndex + 1).byShuntingRegionId;
    | 
    |         % Check if the region ID matches
    |         if byRegionId == i_byRegionId
    |             o_IsExist = true;
    |             return; % Exit the function once a match is found
    |         end
    |     end
    | end
  function o_stBlockDirectionData = BlockDirection_GetData(i_byBlockDirectionId, i_staBlockDirectionArray):
    | function o_stBlockDirectionData = BlockDirection_GetData(i_byBlockDirectionId, i_staBlockDirectionArray)
    |     global g_stStatusCode;
    |     global g_stArrayLens;
    |     % Initialize the index
    |     iIndex = g_stStatusCode.INTDefault;
    | 
    | 
    |    
    |     o_stBlockDirectionData = i_staBlockDirectionArray(1);
    |     % Check if the block direction ID is valid
    |     if i_byBlockDirectionId > g_stStatusCode.MinimumID
    |         % Loop through the block direction array
    |         for iIndex = g_stArrayLens.StartIndex:g_stArrayLens.SendBlockDirectionArrayLen - 1
    |             % Check if the current block direction ID matches the input ID
    |             if i_byBlockDirectionId == i_staBlockDirectionArray(iIndex + 1).byBlockDirectionId
    |                 % Assign the matching block direction data to the output
    |                 o_stBlockDirectionData = i_staBlockDirectionArray(iIndex + 1);
    |             else
    |                 % Not equal ID, do nothing
    |             end
    |         end
    |     else
    |         % Invalid ID, do nothing
    |     end
    | end
  function [o_aPMSetNormalAy, o_aPMSetPowerAy, o_aPMSetReverseAy] = SystemMonitor_SetPointMachineFault:
    | function [o_aPMSetNormalAy, o_aPMSetPowerAy, o_aPMSetReverseAy] = SystemMonitor_SetPointMachineFault()
    | global g_stStatusCode;
    | global g_stArrayLens;
    | global g_stDOModuleAdapter;
    |     % Initialize the index
    |     iIndex = g_stStatusCode.INTDefault;
    |     o_aPMSetNormalAy = false (36,1);
    |     o_aPMSetReverseAy = false (36,1);
    |     o_aPMSetPowerAy = false (36,1);
    |     % Loop through the PointMachineArray
    |     for iIndex = g_stArrayLens.StartIndex:g_stArrayLens.PointMachineArrayLen - 1
    |         % Check if the index is within the bounds of PMSetLen
    |         if iIndex < g_stDOModuleAdapter.PMSetLen
    |             % Set the corresponding elements to IsUnSet
    |             o_aPMSetNormalAy(iIndex + 1) = g_stStatusCode.IsUnSet;
    |             o_aPMSetReverseAy(iIndex + 1) = g_stStatusCode.IsUnSet;
    |             o_aPMSetPowerAy(iIndex + 1) = g_stStatusCode.IsUnSet;
    |         else
    |             % Do nothing if the index is out of bounds
    |         end
    |     end
    | end
  function o_bResult = Shunting_IsSet(i_byRegionId):
    | function o_bResult = Shunting_IsSet(i_byRegionId)
    | 
    |     global g_stStatusCode;
    | 
    |     % 初始化結果為 false
    |     o_bResult = false;
    | 
    |     % 獲取區域數據
    |     stRegionData = Shunting_Get(i_byRegionId);
    | 
    |     % 檢查區域的狀態
    |     if stRegionData.byStatus == g_stStatusCode.IsStatusUnSet
    |         % Shunting 未設置
    |         o_bResult = false;
    |     elseif stRegionData.byStatus == g_stStatusCode.IsStatusSet
    |         % Shunting 已設置
    |         o_bResult = true;
    |     end
    | end
  function o_bResult = SetShunting_CheckSetData(i_byRegionId):
    | function o_bResult = SetShunting_CheckSetData(i_byRegionId)
    |     global g_stErrorCode;
    |     % Initialize the output result
    |     o_bResult = false;
    | 
    |     % Initialize variables
    |     bIsShuntingExist = false;
    |     bIsShuntingTableExist = false;
    | 
    |     % Check shunting data
    |     bIsShuntingExist = CheckData_CheckShuntingData(i_byRegionId);
    | 
    |     % Check shunting region table data
    |     bIsShuntingTableExist = CheckData_CheckShuntingRegionTableData(i_byRegionId);
    | 
    |     % Check if both conditions are true
    |     if bIsShuntingExist && bIsShuntingTableExist
    |         o_bResult = true;
    |     else
    |         o_bResult = false;
    |         
    |         SystemMonitor_SetWarningLog(g_stErrorCode.AH07_01_004);
    |     end
    | end
  function o_stSignalData = Signal_Get(i_bySignalId):
    | function o_stSignalData = Signal_Get(i_bySignalId)
    | global g_staSignal;
    |     o_stSignalData = Signal_GetData(i_bySignalId, g_staSignal);
    | end
  function [o_aSignal1SetAy, o_aSignal2SetAy, o_aSignal3SetAy, o_aSignal4SetAy] = SystemMonitor_SetSignalFault:
    | function [o_aSignal1SetAy, o_aSignal2SetAy, o_aSignal3SetAy, o_aSignal4SetAy] = SystemMonitor_SetSignalFault()
    |     % Initialize the index
    |     global g_stStatusCode;
    |     global g_stArrayLens;
    |     global g_stDOModuleAdapter;
    | 
    |     iIndex = g_stStatusCode.INTDefault;
    |     o_aSignal1SetAy = false(36,1);
    |     o_aSignal2SetAy = false(36,1);
    |     o_aSignal3SetAy = false(36,1);
    |     o_aSignal4SetAy = false(36,1);
    |     % Loop through the SignalArray
    |     for iIndex = g_stArrayLens.StartIndex:g_stArrayLens.SignalArrayLen - 1
    |         % Check if the index is within the bounds of SignalSetAyLen
    |         if iIndex < g_stDOModuleAdapter.SignalSetAyLen
    |             % Set the corresponding elements to IsUnSet
    |             o_aSignal1SetAy(iIndex + 1) = g_stStatusCode.IsUnSet;
    |             o_aSignal2SetAy(iIndex + 1) = g_stStatusCode.IsUnSet;
    |             o_aSignal3SetAy(iIndex + 1) = g_stStatusCode.IsUnSet;
    |             o_aSignal4SetAy(iIndex + 1) = g_stStatusCode.IsUnSet;
    |         else
    |             % Do nothing if the index is out of bounds
    |         end
    |     end
    | end
  function o_bResult = CheckData_CheckShuntingData(i_byRegionId):
    | function o_bResult = CheckData_CheckShuntingData(i_byRegionId)
    |     global g_stStatusCode;
    |     global g_stErrorCode;
    |     % Initialize the output result
    |     o_bResult = false;
    | 
    |     % Initialize variables
    |     bIsShuntingExist = false;
    |     bIsBlockDirectionExist = false;
    |     bIsRoutingExist = false;
    |     bIsTrackExist = false;
    |     bIsSignalExist = false;
    |     bIsPointMachineExist = false;
    |     byBlockDirectionId = g_stStatusCode.BYTEDefault;
    |     
    | 
    |     % Check if shunting exists
    |     bIsShuntingExist = Shunting_IsExist(i_byRegionId);
    | 
    |     if bIsShuntingExist
    |         o_bResult = true;
    | 
    |         % Get shunting region data
    |         stShuntingRegionData = Shunting_Get(i_byRegionId);
    | 
    |         % Get block direction ID
    |         byBlockDirectionId = stShuntingRegionData.byBlockDirectionId;
    | 
    |         % Check if block direction exists
    |         bIsBlockDirectionExist = BlockDirection_IsExist(byBlockDirectionId);
    | 
    |         if ~bIsBlockDirectionExist
    |             o_bResult = false;
    |             SystemMonitor_SetWarningLog(g_stErrorCode.BM10_02_202);
    |         end
    | 
    |         % Check shunting region status
    |         if stShuntingRegionData.byStatus == g_stStatusCode.ShuntingNoneSet || ...
    |            stShuntingRegionData.byStatus == g_stStatusCode.ShuntingIsSet
    |             % Shunting region status is set
    |         else
    |             o_bResult = false;
    |             SystemMonitor_SetWarningLog(g_stErrorCode.BM10_03_217);
    |         end
    | 
    |         % Check data array existence
    |         bIsRoutingExist = CheckData_CheckDataArrayExistLen24(g_stStatusCode.DataTypeRouting, ...
    |                                                           stShuntingRegionData.RoutingIdArray);
    | 
    |         bIsTrackExist = CheckData_CheckDataArrayExistLen8(g_stStatusCode.DataTypeTrack, ...
    |                                                         stShuntingRegionData.TrackIdArray);
    | 
    |         bIsSignalExist = CheckData_CheckDataArrayExistLen8(g_stStatusCode.DataTypeSignal, ...
    |                                                          stShuntingRegionData.SignalIdArray);
    | 
    |         bIsPointMachineExist = CheckData_CheckDataArrayExistLen12(g_stStatusCode.DataTypeSignal, ...
    |                                                                stShuntingRegionData.PointMachineIdArray);
    | 
    |         if ~(bIsRoutingExist && bIsTrackExist && bIsSignalExist && bIsPointMachineExist)
    |             o_bResult = false;
    |             SystemMonitor_SetWarningLog(g_stErrorCode.BM10_04_202);
    |         end
    |     else
    |         o_bResult = false;
    |         SystemMonitor_SetWarningLog(g_stErrorCode.BM10_01_202);
    |     end
    | end
  function Shunting_SetStatus(i_byRegionId, i_bySetCmd):
    | function Shunting_SetStatus(i_byRegionId, i_bySetCmd)
    | global g_stStatusCode;
    | 
    |     stShuntingRegionData = Shunting_Get(i_byRegionId);
    | 
    |     if stShuntingRegionData.byShuntingRegionId > g_stStatusCode.MinimumID
    | 
    |         stShuntingRegionData.byStatus = i_bySetCmd;
    | 
    |         Shunting_Set(i_byRegionId, stShuntingRegionData);
    |     end
    | end
  function SetShunting_SetStatus(i_byRegionId, i_bySetStatus):
    | function SetShunting_SetStatus(i_byRegionId, i_bySetStatus)
    |    global g_stStatusCode;
    | 
    |     % 调用 Shunting_SetStatus
    |     Shunting_SetStatus(i_byRegionId, i_bySetStatus);
    | 
    |     % 调用 Shunting_Get 并更新结构体数据
    |     stShuntingRegionData = Shunting_Get(i_byRegionId);
    | 
    |     % 逻辑判断并调用相应的函数
    |     if i_bySetStatus == true
    |         BlockDirection_SetShunting(stShuntingRegionData.byBlockDirectionId, g_stStatusCode.IsSet);
    |         SetShunting_SetSignalSign(i_byRegionId, g_stStatusCode.IsSet);
    |     else
    |         BlockDirection_SetShunting(stShuntingRegionData.byBlockDirectionId, g_stStatusCode.IsUnSet);
    |         SetShunting_SetSignalSign(i_byRegionId, g_stStatusCode.IsUnSet);
    |     end
    | end
  function o_bResult = CheckData_CheckDataArrayExistLen8(i_byDataType, i_byDataArray):
    | function o_bResult = CheckData_CheckDataArrayExistLen8(i_byDataType, i_byDataArray)
    |     global g_stStatusCode;
    |     global g_stArrayLens;
    |     global g_stErrorCode;
    |     % Initialize variables
    |     o_bResult = true;
    |     iIndex = g_stStatusCode.INTDefault;
    |     byDataArrayId = g_stStatusCode.BYTEDefault;
    |     bIsDataExist = false;
    | 
    |     % Loop through the input array
    |     for iIndex = g_stArrayLens.StartIndex:g_stArrayLens.ArrayLen8 - 1
    |         byDataArrayId = i_byDataArray(iIndex + 1);
    | 
    |         % Check if the data array ID is valid
    |         if byDataArrayId > g_stStatusCode.MinimumID
    |             % Check the existence of the data based on its type
    |             if i_byDataType == g_stStatusCode.DataTypeBlockDirection
    |                 bIsDataExist = BlockDirection_IsExist(byDataArrayId);
    |             elseif i_byDataType == g_stStatusCode.DataTypeLevelCrossing
    |                 bIsDataExist = LevelCrossing_IsExist(byDataArrayId);
    |             elseif i_byDataType == g_stStatusCode.DataTypeMaintenance
    |                 bIsDataExist = Maintenance_IsExist(byDataArrayId);
    |             elseif i_byDataType == g_stStatusCode.DataTypePlatformDoor
    |                 bIsDataExist = PlatformDoor_IsExist(byDataArrayId);
    |             elseif i_byDataType == g_stStatusCode.DataTypePointMachine
    |                 bIsDataExist = PointMachine_IsExist(byDataArrayId);
    |             elseif i_byDataType == g_stStatusCode.DataTypeRouting
    |                 bIsDataExist = Routing_IsExist(byDataArrayId);
    |             elseif i_byDataType == g_stStatusCode.DataTypeShunting
    |                 bIsDataExist = Shunting_IsExist(byDataArrayId);
    |             elseif i_byDataType == g_stStatusCode.DataTypeSignal
    |                 bIsDataExist = Signal_IsExist(byDataArrayId);
    |             elseif i_byDataType == g_stStatusCode.DataTypeStartPoint
    |                 bIsDataExist = StartPoint_IsExist(byDataArrayId);
    |             elseif i_byDataType == g_stStatusCode.DataTypeTrack
    |                 bIsDataExist = Track_IsExist(byDataArrayId);
    |             else
    |                 o_bResult = false; % Data Type not match
    |             end
    | 
    |             % If the data does not exist, set the result to false and log a warning
    |             if ~bIsDataExist
    |                 o_bResult = false;
    |                 SystemMonitor_SetWarningLog(g_stErrorCode.BM01_01_202);
    |             end
    |         end
    |     end
    | end
  function o_stSignalData = Signal_GetData(i_bySignalId, i_staSignalArray):
    | function o_stSignalData = Signal_GetData(i_bySignalId, i_staSignalArray)
    |     global g_stStatusCode;
    |     global g_stArrayLens;
    | 
    |     % 初始化索引
    |     %iIndex = g_stStatusCode.INTDefault;
    | 
    |     o_stSignalData = i_staSignalArray(1);
    |     % 檢查信號 ID 是否大於最小 ID
    |     if i_bySignalId > g_stStatusCode.MinimumID
    |         % 遍歷陣列以查找匹配的信號 ID
    |         for iIndex = g_stArrayLens.StartIndex:g_stArrayLens.SignalArrayLen - 1
    |             if i_bySignalId == i_staSignalArray(iIndex + 1).bySignalId
    |                 o_stSignalData = i_staSignalArray(iIndex + 1);
    |                 return;
    |             end
    |         end
    |     else
    | 
    |     end
    | 
    | end
  function SetShunting_SetSignalSign(i_byRegionId, i_bSetSignalSign):
    | function SetShunting_SetSignalSign(i_byRegionId, i_bSetSignalSign)
    | 
    | global g_stStatusCode;
    | 
    | iIndex = g_stStatusCode.INTDefault;
    | bySignalId = g_stStatusCode.BYTEDefault;
    | bySignalConfig = g_stStatusCode.BYTEDefault;
    | 
    | stShuntingRegionTableData = CheckTable_GetShunting(i_byRegionId);
    | 
    | % 迴圈遍歷 SignalCheckArray
    | for iIndex = g_stArrayLens.StartIndex:(stShuntingRegionTableData.SignalCheckArrayLen - 1)
    | 
    |     bySignalId = stShuntingRegionTableData.SignalCheckArray(iIndex + 1).bySignalId; % MATLAB 索引從 1 開始
    | 
    |     bySignalConfig = stShuntingRegionTableData.SignalCheckArray(iIndex + 1).SignalConfigArray(g_stStatusCode.SignalSignSafeInt + 1).bySignalConfig;
    | 
    |     if bySignalId > g_stStatusCode.MinimumID
    |         if i_bSetSignalSign == true
    |             Signal_SetLightsByConfig(bySignalId, bySignalConfig, g_stStatusCode.SignalSignStop);
    |         else
    |             Signal_SetLightsByConfig(bySignalId, g_stStatusCode.SignalSetConfigInit, g_stStatusCode.SignalLightInit);
    |         end
    |     else
    | 
    |     end
    | end
    | end
  function o_aStartPointAy = SystemMonitor_SetStartPointFault:
    | function o_aStartPointAy = SystemMonitor_SetStartPointFault()
    | global g_stStatusCode;
    | global g_stArrayLens;
    | global g_stDOModuleAdapter;
    |     % Initialize the index
    |     iIndex = g_stStatusCode.INTDefault;
    |     o_aStartPointAy = false(36, 1);
    |     % Loop through the StartPointArray
    |     for iIndex = g_stArrayLens.StartIndex:g_stArrayLens.StartPointArrayLen - 1
    |         % Check if the index is within the bounds of StartPointAyLen
    |         if iIndex < g_stDOModuleAdapter.StartPointAyLen
    |             % Set the corresponding element to IsUnSet
    |             o_aStartPointAy(iIndex + 1) = g_stStatusCode.IsUnSet;
    |         else
    |             % Do nothing if the index is out of bounds
    |         end
    |     end
    | end
  function o_bResult = CheckData_CheckDataArrayExistLen12(i_byDataType, i_byDataArray):
    | function o_bResult = CheckData_CheckDataArrayExistLen12(i_byDataType, i_byDataArray)
    |     global g_stStatusCode;
    |     global g_stArrayLens;
    |     global g_stErrorCode;
    |     % Initialize variables
    |     o_bResult = true;
    |     iIndex = g_stStatusCode.INTDefault;
    |     byDataArrayId = g_stStatusCode.BYTEDefault;
    |     bIsDataExist = false;
    | 
    |     % Loop through the input array
    |     for iIndex = g_stArrayLens.StartIndex:g_stArrayLens.ArrayLen12 - 1
    |         byDataArrayId = i_byDataArray(iIndex + 1);
    | 
    |         % Check if the data array ID is valid
    |         if byDataArrayId > g_stStatusCode.MinimumID
    |             % Check the existence of the data based on its type
    |             if i_byDataType == g_stStatusCode.DataTypeBlockDirection
    |                 bIsDataExist = BlockDirection_IsExist(byDataArrayId);
    |             elseif i_byDataType == g_stStatusCode.DataTypeLevelCrossing
    |                 bIsDataExist = LevelCrossing_IsExist(byDataArrayId);
    |             elseif i_byDataType == g_stStatusCode.DataTypeMaintenance
    |                 bIsDataExist = Maintenance_IsExist(byDataArrayId);
    |             elseif i_byDataType == g_stStatusCode.DataTypePlatformDoor
    |                 bIsDataExist = PlatformDoor_IsExist(byDataArrayId);
    |             elseif i_byDataType == g_stStatusCode.DataTypePointMachine
    |                 bIsDataExist = PointMachine_IsExist(byDataArrayId);
    |             elseif i_byDataType == g_stStatusCode.DataTypeRouting
    |                 bIsDataExist = Routing_IsExist(byDataArrayId);
    |             elseif i_byDataType == g_stStatusCode.DataTypeShunting
    |                 bIsDataExist = Shunting_IsExist(byDataArrayId);
    |             elseif i_byDataType == g_stStatusCode.DataTypeSignal
    |                 bIsDataExist = Signal_IsExist(byDataArrayId);
    |             elseif i_byDataType == g_stStatusCode.DataTypeStartPoint
    |                 bIsDataExist = StartPoint_IsExist(byDataArrayId);
    |             elseif i_byDataType == g_stStatusCode.DataTypeTrack
    |                 bIsDataExist = Track_IsExist(byDataArrayId);
    |             else
    |                 o_bResult = false; % Data Type not match
    |             end
    | 
    |             % If the data does not exist, set the result to false and log a warning
    |             if ~bIsDataExist
    |                 o_bResult = false;
    |                 SystemMonitor_SetWarningLog(g_stErrorCode.BM01_01_202);
    |             end
    |         end
    |     end
    | end
  function o_bResult = Routing_IsExist(i_byRoutingId):
    | function o_bResult = Routing_IsExist(i_byRoutingId)
    |     global g_stStatusCode;  
    |     o_bResult = CheckData_CheckDataExist(g_stStatusCode.DataTypeRouting, i_byRoutingId);
    | end
  function o_bResult = StartPoint_IsExist(i_byStartPointId):
    | function o_bResult = StartPoint_IsExist(i_byStartPointId)
    |    global g_stStatusCode;
    |    o_bResult = CheckData_CheckDataExist(g_stStatusCode.DataTypeStartPoint, i_byStartPointId);
    | end
  function o_bResult = LevelCrossing_IsExist(i_byCrossingId):
    | function o_bResult = LevelCrossing_IsExist(i_byCrossingId)
    |    global g_stStatusCode;
    |    o_bResult = CheckData_CheckDataExist(g_stStatusCode.DataTypeLevelCrossing, i_byCrossingId);
    | end
  function o_bResult = Track_IsExist(i_byTrackId):
    | function o_bResult = Track_IsExist(i_byTrackId)
    |     global g_stStatusCode;
    |     o_bResult = false;
    |     o_bResult = CheckData_CheckDataExist(g_stStatusCode.DataTypeTrack, i_byTrackId); 
    | end
  function o_bResult = PlatformDoor_IsExist(i_byDoorId):
    | function o_bResult = PlatformDoor_IsExist(i_byDoorId)
    |     global g_stStatusCode;
    |     o_bResult = CheckData_CheckDataExist(g_stStatusCode.DataTypePlatformDoor, i_byDoorId);
    | end
  function o_bResult = Signal_IsExist(i_bySignalId):
    | function o_bResult = Signal_IsExist(i_bySignalId)
    |     global g_stStatusCode;
    |     o_bResult = CheckData_CheckDataExist(g_stStatusCode.DataTypeSignal, i_bySignalId);
    | end
  function CommonCommand_Complete(i_bCommandStatus):
    | function CommonCommand_Complete(i_bCommandStatus)
    |     global g_stExecuteIXLCommand;
    |     % Set the status of ExecuteIXLCommand
    |     g_stExecuteIXLCommand.byStatus = i_bCommandStatus;
    | end
  function o_aTrackResetAy = SystemMonitor_SetTrackFault:
    | function o_aTrackResetAy = SystemMonitor_SetTrackFault()
    | global g_stStatusCode;
    | global g_stArrayLens;
    | global g_stDOModuleAdapter;
    |     % Initialize the index
    |     iIndex = g_stStatusCode.INTDefault;
    |     o_aTrackResetAy = false(48, 1);
    |     % Loop through the TrackArray
    |     for iIndex = g_stArrayLens.StartIndex:g_stArrayLens.TrackArrayLen - 1
    |         % Check if the index is within the bounds of TrackResetAyLen
    |         if iIndex < g_stDOModuleAdapter.TrackResetAyLen
    |             % Set the corresponding element to IsUnSet
    |             o_aTrackResetAy(iIndex + 1) = g_stStatusCode.IsUnSet;
    |         else
    |             % Do nothing if the index is out of bounds
    |         end
    |     end
    | end
  function o_bResult = CheckData_CheckDataArrayExistLen24(i_byDataType, i_byDataArray):
    | function o_bResult = CheckData_CheckDataArrayExistLen24(i_byDataType, i_byDataArray)
    |     global g_stStatusCode;
    |     global g_stArrayLens;
    |     global g_stErrorCode;
    |     % Initialize variables
    |     o_bResult = true;
    |     iIndex = g_stStatusCode.INTDefault;
    |     byDataArrayId = g_stStatusCode.BYTEDefault;
    |     bIsDataExist = false;
    | 
    |     % Loop through the input array
    |     for iIndex = g_stArrayLens.StartIndex:g_stArrayLens.ArrayLen24 - 1
    |         byDataArrayId = i_byDataArray(iIndex + 1);
    | 
    |         % Check if the data array ID is valid
    |         if byDataArrayId > g_stStatusCode.MinimumID
    |             % Check the existence of the data based on its type
    |             if i_byDataType == g_stStatusCode.DataTypeBlockDirection
    |                 bIsDataExist = BlockDirection_IsExist(byDataArrayId);
    |             elseif i_byDataType == g_stStatusCode.DataTypeLevelCrossing
    |                 bIsDataExist = LevelCrossing_IsExist(byDataArrayId);
    |             elseif i_byDataType == g_stStatusCode.DataTypeMaintenance
    |                 bIsDataExist = Maintenance_IsExist(byDataArrayId);
    |             elseif i_byDataType == g_stStatusCode.DataTypePlatformDoor
    |                 bIsDataExist = PlatformDoor_IsExist(byDataArrayId);
    |             elseif i_byDataType == g_stStatusCode.DataTypePointMachine
    |                 bIsDataExist = PointMachine_IsExist(byDataArrayId);
    |             elseif i_byDataType == g_stStatusCode.DataTypeRouting
    |                 bIsDataExist = Routing_IsExist(byDataArrayId);
    |             elseif i_byDataType == g_stStatusCode.DataTypeShunting
    |                 bIsDataExist = Shunting_IsExist(byDataArrayId);
    |             elseif i_byDataType == g_stStatusCode.DataTypeSignal
    |                 bIsDataExist = Signal_IsExist(byDataArrayId);
    |             elseif i_byDataType == g_stStatusCode.DataTypeStartPoint
    |                 bIsDataExist = StartPoint_IsExist(byDataArrayId);
    |             elseif i_byDataType == g_stStatusCode.DataTypeTrack
    |                 bIsDataExist = Track_IsExist(byDataArrayId);
    |             else
    |                 o_bResult = false; % Data Type not match
    |             end
    | 
    |             % If the data does not exist, set the result to false and log a warning
    |             if ~bIsDataExist
    |                 o_bResult = false;
    |                 SystemMonitor_SetWarningLog(g_stErrorCode.BM01_01_202);
    |             end
    |         end
    |     end
    | end
  function o_bResult = Routing_IsExecute(i_byRoutingId):
    | function o_bResult = Routing_IsExecute(i_byRoutingId)
    | global g_stStatusCode;
    | 
    |     stRoutingData = Routing_Get(i_byRoutingId);
    | 
    |     if stRoutingData.byRoutingId == g_stStatusCode.MinimumID
    |         
    |         if stRoutingData.byStatus == g_stStatusCode.RoutingNone
    | 
    |             o_bResult = false;
    |         else
    |             o_bResult = true; 
    |         end
    |     else  
    |         o_bResult = true;
    |     end
    | 
    | end
  function o_bResult = Signal_IsLock(i_bySignalId):
    | function o_bResult = Signal_IsLock(i_bySignalId)
    | 
    |     % 初始化結果為 false
    |     o_bResult = false;
    | 
    |     % 獲取信號數據
    |     stSignalData = Signal_Get(i_bySignalId);
    | 
    |     % 設置結果
    |     o_bResult = stSignalData.bIsLock;
    | end
  function CommonCommand_Discard(i_bCommandStatus):
    | function CommonCommand_Discard(i_bCommandStatus)
    |  % Set the status of ExecuteIXLCommand
    |  
    |     global g_stExecuteIXLCommand;
    |    
    | 
    | 
    | 
    | 
    | 
    |     g_stExecuteIXLCommand.byStatus = i_bCommandStatus;
    | 
    | end
  function o_bResult = CheckData_CheckDataExist(i_byDataType, i_byDataId):
    | function o_bResult = CheckData_CheckDataExist(i_byDataType, i_byDataId)
    |     global g_stStatusCode;
    |     global g_stArrayLens;
    |     global g_staSendBlockDirection;
    |     global g_staLevelCrossing;
    |     global g_staMaintenanceRegion;
    |     global g_staPlatformDoor;
    |     global g_staPointMachine;
    |     global g_staRouting;
    |     global g_staShuntingRegion;
    |     global g_staSignal;
    |     global g_staStartPoint;
    |     global g_staTrack;
    |     global g_staSignalTruthTable;
    |     %Initialize the output result
    |     o_bResult = false;
    | 
    |     % Initialize variables
    |     iIndex = g_stStatusCode.INTDefault;
    |     iDataLen = g_stStatusCode.INTDefault;
    |     byDataId = g_stStatusCode.BYTEDefault;
    | 
    |     % Check if the data ID is greater than the minimum ID
    |     if i_byDataId > g_stStatusCode.MinimumID
    |         % Get the data array length
    |         iDataLen = CheckData_GetDataArrayLen(i_byDataType);
    | 
    |         % Loop through the data array
    |         for iIndex = g_stArrayLens.StartIndex:(iDataLen -1)
    |         %for iIndex = g_stArrayLens.StartIndex:g_stArrayLens.StartIndex
    |             % Determine the data ID based on the data type
    |             if i_byDataType == g_stStatusCode.DataTypeBlockDirection
    |                 byDataId = g_staSendBlockDirection(iIndex + 1).byBlockDirectionId;
    |             elseif i_byDataType == g_stStatusCode.DataTypeLevelCrossing
    |                 byDataId = g_staLevelCrossing(iIndex + 1).byCrossingId;
    |             elseif i_byDataType == g_stStatusCode.DataTypeMaintenance
    |                 byDataId = g_staMaintenanceRegion(iIndex + 1).byMaintenanceRegionId;
    |             elseif i_byDataType == g_stStatusCode.DataTypePlatformDoor
    |                 byDataId = g_staPlatformDoor(iIndex + 1).byDoorId;
    |             elseif i_byDataType == g_stStatusCode.DataTypePointMachine
    |                 byDataId = g_staPointMachine(iIndex + 1).byPointMachineId;
    |             elseif i_byDataType == g_stStatusCode.DataTypeRouting
    |                 byDataId = g_staRouting(iIndex + 1).byRoutingId;
    |             elseif i_byDataType == g_stStatusCode.DataTypeShunting
    |                 byDataId = g_staShuntingRegion(iIndex + 1).byShuntingRegionId;
    |             elseif i_byDataType == g_stStatusCode.DataTypeSignal
    |                 byDataId = g_staSignal(iIndex + 1).bySignalId;
    |             elseif i_byDataType == g_stStatusCode.DataTypeStartPoint
    |                 byDataId = g_staStartPoint(iIndex + 1).byStartPointId;
    |             elseif i_byDataType == g_stStatusCode.DataTypeTrack
    |                 byDataId = g_staTrack(iIndex + 1).byTrackId;
    |             elseif i_byDataType == g_stStatusCode.DataTypeSignalTruthTable
    |                 byDataId = g_staSignalTruthTable(iIndex + 1).bySignalConfig;
    |             else
    |                 byDataId = g_stStatusCode.BYTEDefault; % DataType not match
    |             end
    | 
    |             % Check if the data ID matches
    |             if i_byDataId == byDataId
    |                 o_bResult = true;
    |                 break;
    |             end
    |         end
    |     end
    | end
  function o_stRoutingData = Routing_Get(i_byRoutingId):
    | function o_stRoutingData = Routing_Get(i_byRoutingId)
    | global g_staRouting;
    | o_stRoutingData = Routing_GetData(i_byRoutingId, g_staRouting);
    | end
  function o_iDataArrayLen = CheckData_GetDataArrayLen(i_byDataType):
    | function o_iDataArrayLen = CheckData_GetDataArrayLen(i_byDataType)
    |     global g_stStatusCode;
    |     global g_stArrayLens;
    |     % Initialize the output length
    |     %o_iDataArrayLen = g_stStatusCode.INTDefault;
    | 
    |     % Determine the data array length based on the data type
    |     if i_byDataType == g_stStatusCode.DataTypeBlockDirection
    |         o_iDataArrayLen = g_stArrayLens.SendBlockDirectionArrayLen;
    |     elseif i_byDataType == g_stStatusCode.DataTypeLevelCrossing
    |         o_iDataArrayLen = g_stArrayLens.LevelCrossingArrayLen;
    |     elseif i_byDataType == g_stStatusCode.DataTypeMaintenance
    |         o_iDataArrayLen = g_stArrayLens.MaintenanceRegionArrayLen;
    |     elseif i_byDataType == g_stStatusCode.DataTypePlatformDoor
    |         o_iDataArrayLen = g_stArrayLens.PlatformDoorArrayLen;
    |     elseif i_byDataType == g_stStatusCode.DataTypePointMachine
    |         o_iDataArrayLen = g_stArrayLens.PointMachineArrayLen;
    |     elseif i_byDataType == g_stStatusCode.DataTypeRouting
    |         o_iDataArrayLen = g_stArrayLens.RoutingArrayLen;
    |     elseif i_byDataType == g_stStatusCode.DataTypeShunting
    |         o_iDataArrayLen = g_stArrayLens.ShuntingRegionArrayLen;
    |     elseif i_byDataType == g_stStatusCode.DataTypeSignal
    |         o_iDataArrayLen = g_stArrayLens.SignalArrayLen;
    |     elseif i_byDataType == g_stStatusCode.DataTypeStartPoint
    |         o_iDataArrayLen = g_stArrayLens.StartPointArrayLen;
    |     elseif i_byDataType == g_stStatusCode.DataTypeTrack
    |         o_iDataArrayLen = g_stArrayLens.TrackArrayLen;
    |     elseif i_byDataType == g_stStatusCode.DataTypeSignalTruthTable
    |         o_iDataArrayLen = g_stArrayLens.SignalTruthTableArrayLen;
    |     else
    |         o_iDataArrayLen = g_stStatusCode.INTDefault; % Data Type not match
    |     end
    | end
  function SystemMonitor_SetSafeLog(i_uliErrorCodeUid):
    | function SystemMonitor_SetSafeLog(i_uliErrorCodeUid)
    |     global g_stStatusCode;
    |     % Set the log with the error code and safe type
    |     SystemMonitor_SetLog(i_uliErrorCodeUid, g_stStatusCode.ErrorCodeSafeType);
    | end
  function Signal_SetLightsByConfig(i_bySignalId, i_bySignalConfig, i_bySignalSign):
    | function Signal_SetLightsByConfig(i_bySignalId, i_bySignalConfig, i_bySignalSign)
    |    
    |     
    |     stSignalData = Signal_Get(i_bySignalId); 
    |     
    |     [bLight1, bLight2, bLight3, bLight4] = Signal_GetLightsByConfig(i_bySignalConfig);
    |     
    |     stSignalData.bSetLight1 = bLight1;
    |     stSignalData.bSetLight2 = bLight2;
    |     stSignalData.bSetLight3 = bLight3;
    |     stSignalData.bSetLight4 = bLight4;
    |     stSignalData.bySetConfig = i_bySignalConfig;
    |     stSignalData.bySignalSign = i_bySignalSign;
    |     
    |     Signal_Set(i_bySignalId, stSignalData);
    | end
  function o_stRoutingData = Routing_GetData(i_byRoutingId, i_staRoutingArray):
    | function o_stRoutingData = Routing_GetData(i_byRoutingId, i_staRoutingArray)
    |     global g_stStatusCode;
    |     global g_stArrayLens;
    |     
    |     
    |     o_stRoutingData = i_staRoutingArray(1);
    |     % 檢查區域 ID 是否大於最小 ID
    |     if i_byRoutingId > g_stStatusCode.MinimumID
    |         % 遍歷陣列以查找匹配的區域 ID
    |         for iIndex = g_stArrayLens.StartIndex:g_stArrayLens.RoutingArrayLen - 1
    |             if i_byRoutingId == i_staRoutingArray(iIndex + 1).byRoutingId
    |                 o_stRoutingData = i_staRoutingArray(iIndex + 1);
    |                 return;
    |             end
    |         end
    |     else
    |         
    |     end
    | 
    | end
  function SystemMonitor_SetWarningLog(i_uliErrorCodeUid):
    | function SystemMonitor_SetWarningLog(i_uliErrorCodeUid)
    |     global g_stStatusCode;
    |     SystemMonitor_SetLog(i_uliErrorCodeUid, g_stStatusCode.ErrorCodeWarningType);
    | end
  function [o_bLight1, o_bLight2, o_bLight3, o_bLight4] = Signal_GetLightsByConfig(i_bySignalConfig):
    | function [o_bLight1, o_bLight2, o_bLight3, o_bLight4] = Signal_GetLightsByConfig(i_bySignalConfig)
    | 
    | global g_staSignalTruthTable;
    | 
    | [o_bLight1, o_bLight2, o_bLight3, o_bLight4] = Signal_GetLightsByConfigData(i_bySignalConfig, g_staSignalTruthTable);
    | end
  function o_stPointMachineData = PointMachine_Get(i_byPointMachineId):
    | function o_stPointMachineData = PointMachine_Get(i_byPointMachineId)
    | global g_staPointMachine;
    |     o_stPointMachineData = PointMachine_GetData(i_byPointMachineId, g_staPointMachine);
    | end
  function SystemMonitor_SetErrorLog(i_uliErrorCodeUid):
    | function SystemMonitor_SetErrorLog(i_uliErrorCodeUid)
    |     global g_stStatusCode;
    |     % Set the error log with the error code and error type
    |     SystemMonitor_SetLog(i_uliErrorCodeUid, g_stStatusCode.ErrorCodeErrorType);
    | end
  function [o_bLight1, o_bLight2, o_bLight3, o_bLight4] = Signal_GetLightsByConfigData(i_bySignalConfig, i_staSignalTruthTableArray):
    | function [o_bLight1, o_bLight2, o_bLight3, o_bLight4] = Signal_GetLightsByConfigData(i_bySignalConfig, i_staSignalTruthTableArray)
    |     
    | global g_stStatusCode g_stArrayLens; % 如果需要全局變數
    |     
    |     o_bLight1 = false;
    |     o_bLight2 = false;
    |     o_bLight3 = false;
    |     o_bLight4 = false;
    |     
    |     for iIndex = g_stArrayLens.StartIndex:g_stArrayLens.SignalTruthTableArrayLen-1
    |         bySignalConfig = i_staSignalTruthTableArray(iIndex+1).bySignalConfig; 
    |         
    |         if (bySignalConfig == i_bySignalConfig && i_staSignalTruthTableArray(iIndex+1).byTruthTableId > g_stStatusCode.MinimumID)
    |             o_bLight1 = i_staSignalTruthTableArray(iIndex+1).bLight1;
    |             o_bLight2 = i_staSignalTruthTableArray(iIndex+1).bLight2;
    |             o_bLight3 = i_staSignalTruthTableArray(iIndex+1).bLight3;
    |             o_bLight4 = i_staSignalTruthTableArray(iIndex+1).bLight4;
    |         else
    |             bySignalConfig = g_stStatusCode.BYTEDefault;
    |         end
    |     end
    | end
  function ReportMonitor_SystemValue:
    | function ReportMonitor_SystemValue()
    | global g_stOpcuaAdapter;
    | global g_stSystemValue;
    |     % Assign values from SystemValue to OpcuaAdapter
    |     g_stOpcuaAdapter.SystemValue.IsInit = g_stSystemValue.IsInit;
    |     g_stOpcuaAdapter.SystemValue.byProgramStatus = g_stSystemValue.byProgramStatus;
    |     g_stOpcuaAdapter.SystemValue.Timestamp_ms = g_stSystemValue.Timestamp_ms;
    |     g_stOpcuaAdapter.SystemValue.Timestamp_sec = g_stSystemValue.Timestamp_sec;
    | end
  function o_stPointMachineData = PointMachine_GetData(i_byPointMachineId, i_staPointMachineArray):
    | function o_stPointMachineData = PointMachine_GetData(i_byPointMachineId, i_staPointMachineArray)
    |     global g_stStatusCode;
    |     global g_stArrayLens;
    |     % 初始化索引
    |     %iIndex = g_stStatusCode.INTDefault;
    | 
    |     o_stPointMachineData = i_staPointMachineArray(1);
    |     % 檢查 Point Machine ID 是否大於最小 ID
    |     if i_byPointMachineId > g_stStatusCode.MinimumID
    |         % 遍歷陣列以查找匹配的 Point Machine ID
    |         for iIndex = g_stArrayLens.StartIndex:g_stArrayLens.PointMachineArrayLen - 1
    |             if i_byPointMachineId == i_staPointMachineArray(iIndex + 1).byPointMachineId
    |                 o_stPointMachineData = i_staPointMachineArray(iIndex + 1);
    |                 return;
    |             end
    |         end
    |     else
    |   
    |     end
    | end
  function SystemMonitor_SetProgramException(i_uliErrorCodeUid):
    | function SystemMonitor_SetProgramException(i_uliErrorCodeUid)
    |     global g_stSystemValue;
    |     global g_stStatusCode;
    |     % Set the program status to exception
    |     g_stSystemValue.byProgramStatus = g_stStatusCode.SystemValueProgramStatusException;
    | 
    |     % Set the error log
    |     SystemMonitor_SetErrorLog(i_uliErrorCodeUid);
    | end
  function Signal_Set(i_bySignalId, i_stSignalData):
    | function Signal_Set(i_bySignalId, i_stSignalData)
    |     
    | global g_staSignal;    
    | 
    |     % Set the block direction data
    |     staSignalAy = Signal_SetData(i_bySignalId, i_stSignalData, g_staSignal);
    | 
    |     % Copy the array
    |     g_staSignal = staSignalAy;
    | end
  function o_bResult = PointMachine_IsPositionCorrect(i_byPointMachineId, i_byPointMachinePosition):
    | function o_bResult = PointMachine_IsPositionCorrect(i_byPointMachineId, i_byPointMachinePosition)
    |     global g_stStatusCode;
    |     
    |     % 初始化結果為 false
    |     o_bResult = false;
    | 
    |     % 獲取 Point Machine 數據
    |     stPointMachineData = PointMachine_Get(i_byPointMachineId);
    | 
    |     % 檢查位置是否正確
    |     if ~stPointMachineData.bNormal && stPointMachineData.bReverse && i_byPointMachinePosition == g_stStatusCode.PointMachinePositionReverse
    |         o_bResult = true;
    |     elseif stPointMachineData.bNormal && ~stPointMachineData.bReverse && i_byPointMachinePosition == g_stStatusCode.PointMachinePositionNormal
    |         o_bResult = true;
    |     else
    |         o_bResult = false;
    |     end
    | end
  function ReportObject_MaintenanceRegionST:
    | function ReportObject_MaintenanceRegionST()
    | global g_stStatusCode;
    | global g_stArrayLens;
    | global g_stOpcuaAdapter;
    | global g_staMaintenanceRegion;
    |     % Initialize index
    |     iIndex = g_stStatusCode.INTDefault;
    | 
    |     % Loop through the array
    |     for iIndex = g_stArrayLens.StartIndex:g_stOpcuaAdapter.ReportMaintenanceRegionArrayLen - 1
    |         if iIndex < g_stArrayLens.MaintenanceRegionArrayLen
    |             if g_staMaintenanceRegion(iIndex + 1).byMaintenanceRegionId > g_stStatusCode.MinimumID
    |                 % Assign values to OpcuaAdapter
    |                 g_stOpcuaAdapter.ReportMaintenanceRegionArray(iIndex + 1).byMaintenanceRegionId = ...
    |                     g_staMaintenanceRegion(iIndex + 1).byMaintenanceRegionId;
    |                 g_stOpcuaAdapter.ReportMaintenanceRegionArray(iIndex + 1).byStatus = ...
    |                     g_staMaintenanceRegion(iIndex + 1).byStatus;
    |             else
    |                 % Invalid ID (no action needed)
    |             end
    |         else
    |             % Over MaintenanceRegionArray size (no action needed)
    |         end
    |     end
    | end
  function SystemMonitor_SetLog(i_uliErrorCodeUid, i_byType):
    | function SystemMonitor_SetLog(i_uliErrorCodeUid, i_byType)
    |     global g_stSystemValue;
    |     global g_staErrorData;
    |     global g_stArrayLens;
    |     % Check if the error count is within the allowed range
    |     if g_stSystemValue.ErrorCount < g_stArrayLens.ErrorDataLen
    |         % Set the error ID and type in the ErrorDataArray
    |         g_staErrorData(g_stSystemValue.ErrorCount + 1).ErrorId = i_uliErrorCodeUid;
    |         g_staErrorData(g_stSystemValue.ErrorCount + 1).ErrorType = i_byType;
    | 
    |         % Increment the error count
    |         g_stSystemValue.ErrorCount = g_stSystemValue.ErrorCount + 1;
    |     else
    |         % Error count exceeds the buffer length, do nothing
    |     end
    | end
  function o_bResult = PointMachine_IsExist(i_byPointMachineId):
    | function o_bResult = PointMachine_IsExist(i_byPointMachineId)
    |    global g_stStatusCode;
    |    o_bResult = CheckData_CheckDataExist(g_stStatusCode.DataTypePointMachine, i_byPointMachineId);
    | end
  function o_staSignalArray = Signal_SetData(i_bySignalId, i_stSignalData, i_staSignalArray):
    | function o_staSignalArray = Signal_SetData(i_bySignalId, i_stSignalData, i_staSignalArray)
    |     global g_stStatusCode;
    |     global g_stArrayLens;
    |     % Initialize the index
    |    
    |     o_staSignalArray = i_staSignalArray;
    |     % Check if the region ID is valid
    |     if i_bySignalId > g_stStatusCode.MinimumID
    |         % Loop through the shunting region array
    |         for iIndex = g_stArrayLens.StartIndex:(g_stArrayLens.SignalArrayLen - 1)
    |             if i_bySignalId == o_staSignalArray(iIndex + 1).bySignalId
    |                 % Update the shunting region data
    |                 o_staSignalArray(iIndex + 1) = i_stSignalData;
    |             else
    |                 % Not equal ID, do nothing
    |             end
    |         end
    |     else
    |         % Invalid ID, do nothing
    |     end
    | end
  function ReportObject_PointMachineST:
    | function ReportObject_PointMachineST()
    | global g_stStatusCode;
    | global g_stArrayLens;
    | global g_stOpcuaAdapter;
    | global g_staPointMachine;
    |     % Initialize index
    |     iIndex = g_stStatusCode.INTDefault;
    | 
    |     % Loop through the array
    |     for iIndex = g_stArrayLens.StartIndex:g_stOpcuaAdapter.ReportPointMachineArrayLen - 1
    |         if iIndex < g_stArrayLens.PointMachineArrayLen
    |             if g_staPointMachine(iIndex + 1).byPointMachineId > g_stStatusCode.MinimumID
    |                 % Assign values to OpcuaAdapter
    |                 g_stOpcuaAdapter.ReportPointMachineArray(iIndex + 1).byPointMachineId = ...
    |                     g_staPointMachine(iIndex + 1).byPointMachineId;
    |                 g_stOpcuaAdapter.ReportPointMachineArray(iIndex + 1).bNormal = ...
    |                     g_staPointMachine(iIndex + 1).bNormal;
    |                 g_stOpcuaAdapter.ReportPointMachineArray(iIndex + 1).bReverse = ...
    |                     g_staPointMachine(iIndex + 1).bReverse;
    |                 g_stOpcuaAdapter.ReportPointMachineArray(iIndex + 1).bPower = ...
    |                     g_staPointMachine(iIndex + 1).bPower;
    |                 g_stOpcuaAdapter.ReportPointMachineArray(iIndex + 1).bLock = ...
    |                     g_staPointMachine(iIndex + 1).bLock;
    |                 g_stOpcuaAdapter.ReportPointMachineArray(iIndex + 1).bException = ...
    |                     g_staPointMachine(iIndex + 1).bException;
    |                 g_stOpcuaAdapter.ReportPointMachineArray(iIndex + 1).bChannelFault = ...
    |                     g_staPointMachine(iIndex + 1).bChannelFault;
    |                 g_stOpcuaAdapter.ReportPointMachineArray(iIndex + 1).bManual = ...
    |                     g_staPointMachine(iIndex + 1).bManual;
    |             else
    |                 % Invalid ID (no action needed)
    |             end
    |         else
    |             % Over PointMachineArray size (no action needed)
    |         end
    |     end
    | end
  function SystemMonitor_ResetErrorLog:
    | function SystemMonitor_ResetErrorLog()
    | global g_stStatusCode;
    | global g_stSystemValue;
    | global g_stArrayLens;
    | global g_staErrorData;
    | 
    |     % Initialize the index
    |     iIndex = g_stStatusCode.INTDefault;
    | 
    |     % Reset the error count
    |     g_stSystemValue.ErrorCount = g_stStatusCode.StartCount;
    | 
    |     % Loop through the ErrorDataArray
    |     for iIndex = g_stArrayLens.StartIndex:g_stArrayLens.ErrorDataLen - 1
    |         % Reset the ErrorId and ErrorType fields
    |         g_staErrorData(iIndex + 1).ErrorId = g_stStatusCode.ULINTDefault;
    |         g_staErrorData(iIndex + 1).ErrorType = g_stStatusCode.ErrorCodeInitType;
    |     end
    | end
  function ReportObject_RoutingST:
    | function ReportObject_RoutingST()
    | global g_stStatusCode;
    | global g_stArrayLens;
    | global g_stOpcuaAdapter;
    | global g_staRouting;
    |     % Initialize index
    |     iIndex = g_stStatusCode.INTDefault;
    | 
    |     % Loop through the array
    |     for iIndex = g_stArrayLens.StartIndex:g_stOpcuaAdapter.ReportRoutingArrayLen - 1
    |         if iIndex < g_stArrayLens.RoutingArrayLen
    |             if g_staRouting(iIndex + 1).byRoutingId > g_stStatusCode.MinimumID
    |                 % Assign values to OpcuaAdapter
    |                 g_stOpcuaAdapter.ReportRoutingArray(iIndex + 1).byRoutingId = ...
    |                     g_staRouting(iIndex + 1).byRoutingId;
    |                 g_stOpcuaAdapter.ReportRoutingArray(iIndex + 1).byFrom = ...
    |                     g_staRouting(iIndex + 1).byFrom;
    |                 g_stOpcuaAdapter.ReportRoutingArray(iIndex + 1).byTo = ...
    |                     g_staRouting(iIndex + 1).byTo;
    |                 g_stOpcuaAdapter.ReportRoutingArray(iIndex + 1).byStatus = ...
    |                     g_staRouting(iIndex + 1).byStatus;
    |             else
    |                 % Invalid ID (no action needed)
    |             end
    |         else
    |             % Over RoutingArray size (no action needed)
    |         end
    |     end
    | end
  function ReportObject_ShuntingRegionST:
    | function ReportObject_ShuntingRegionST()
    | global g_stStatusCode;
    | global g_stArrayLens;
    | global g_stOpcuaAdapter;
    | global g_staShuntingRegion;
    |     % Initialize index
    |     iIndex = g_stStatusCode.INTDefault;
    | 
    |     % Loop through the array
    |     for iIndex = g_stArrayLens.StartIndex:(g_stOpcuaAdapter.ReportShuntingRegionArrayLen - 1)
    |         if iIndex < g_stArrayLens.ShuntingRegionArrayLen
    |             if g_staShuntingRegion(iIndex + 1).byShuntingRegionId > g_stStatusCode.MinimumID
    |                 % Assign values to OpcuaAdapter
    |                 g_stOpcuaAdapter.ReportShuntingRegionArray(iIndex + 1).byShuntingRegionId = ...
    |                     g_staShuntingRegion(iIndex + 1).byShuntingRegionId;
    |                 g_stOpcuaAdapter.ReportShuntingRegionArray(iIndex + 1).byStatus = ...
    |                     g_staShuntingRegion(iIndex + 1).byStatus;
    |             else
    |                 % Invalid ID (no action needed)
    |             end
    |         else
    |             % Over ShuntingRegionArray size (no action needed)
    |         end
    |     end
    | end
  function ReportObject_SignalST:
    | function ReportObject_SignalST()
    | global g_stStatusCode;
    | global g_stArrayLens;
    | global g_stOpcuaAdapter;
    | global g_staSignal;
    |     % Initialize index
    |     iIndex = g_stStatusCode.INTDefault;
    | 
    |     % Loop through the array
    |     for iIndex = g_stArrayLens.StartIndex:(g_stOpcuaAdapter.ReportSignalArrayLen - 1)
    |         if iIndex < g_stArrayLens.SignalArrayLen
    |             if g_staSignal(iIndex + 1).bySignalId > g_stStatusCode.MinimumID
    |                 % Assign values to OpcuaAdapter
    |                 g_stOpcuaAdapter.ReportSignalArray(iIndex + 1).bySignalId = ...
    |                     g_staSignal(iIndex + 1).bySignalId;
    |                 g_stOpcuaAdapter.ReportSignalArray(iIndex + 1).bLight1 = ...
    |                     g_staSignal(iIndex + 1).bLight1;
    |                 g_stOpcuaAdapter.ReportSignalArray(iIndex + 1).bLight2 = ...
    |                     g_staSignal(iIndex + 1).bLight2;
    |                 g_stOpcuaAdapter.ReportSignalArray(iIndex + 1).bLight3 = ...
    |                     g_staSignal(iIndex + 1).bLight3;
    |                 g_stOpcuaAdapter.ReportSignalArray(iIndex + 1).bLight4 = ...
    |                     g_staSignal(iIndex + 1).bLight4;
    |                 g_stOpcuaAdapter.ReportSignalArray(iIndex + 1).bLock = ...
    |                     g_staSignal(iIndex + 1).bIsLock;
    |                 g_stOpcuaAdapter.ReportSignalArray(iIndex + 1).bException = ...
    |                     g_staSignal(iIndex + 1).bException;
    |                 g_stOpcuaAdapter.ReportSignalArray(iIndex + 1).bChannelFault = ...
    |                     g_staSignal(iIndex + 1).bChannelFault;
    |             else
    |                 % Invalid ID (no action needed)
    |             end
    |         else
    |             % Over SignalArray size (no action needed)
    |         end
    |     end
    | end
  function ReportObject_TrackST:
    | function ReportObject_TrackST()
    | global g_stStatusCode;
    | global g_stArrayLens;
    | global g_stOpcuaAdapter;
    | global g_staTrack;
    |     % Initialize index
    |     iIndex = g_stStatusCode.INTDefault;
    | 
    |     % Loop through the array
    |     for iIndex = g_stArrayLens.StartIndex:g_stOpcuaAdapter.ReportTrackArrayLen - 1
    |         if iIndex < g_stArrayLens.TrackArrayLen
    |             if g_staTrack(iIndex + 1).byTrackId > g_stStatusCode.MinimumID
    |                 % Assign values to OpcuaAdapter
    |                 g_stOpcuaAdapter.ReportTrackArray(iIndex + 1).byTrackId = ...
    |                     g_staTrack(iIndex + 1).byTrackId;
    |                 g_stOpcuaAdapter.ReportTrackArray(iIndex + 1).bOccupy = ...
    |                     g_staTrack(iIndex + 1).bOccupy;
    |                 g_stOpcuaAdapter.ReportTrackArray(iIndex + 1).bDisturbed = ...
    |                     g_staTrack(iIndex + 1).bDisturbed;
    |                 g_stOpcuaAdapter.ReportTrackArray(iIndex + 1).bFree = ...
    |                     g_staTrack(iIndex + 1).bFree;
    |                 g_stOpcuaAdapter.ReportTrackArray(iIndex + 1).bSet = ...
    |                     g_staTrack(iIndex + 1).bSet;
    |                 g_stOpcuaAdapter.ReportTrackArray(iIndex + 1).bLock = ...
    |                     g_staTrack(iIndex + 1).bLock;
    |                 g_stOpcuaAdapter.ReportTrackArray(iIndex + 1).bReset = ...
    |                     g_staTrack(iIndex + 1).bReset;
    |                 g_stOpcuaAdapter.ReportTrackArray(iIndex + 1).bException = ...
    |                     g_staTrack(iIndex + 1).bException;
    |                 g_stOpcuaAdapter.ReportTrackArray(iIndex + 1).bChannelFault = ...
    |                     g_staTrack(iIndex + 1).bChannelFault;
    |             else
    |                 % Invalid ID (no action needed)
    |             end
    |         else
    |             % Over TrackArray size (no action needed)
    |         end
    |     end
    | end
